simulink model "Solo_fast_2"  (R2024b)
settings: Solver=VariableStepAuto  StartTime=0.0  StopTime=86400*2  RelTol=1e-3
settings Model: Creator=Laura  LastModifiedBy=Laura

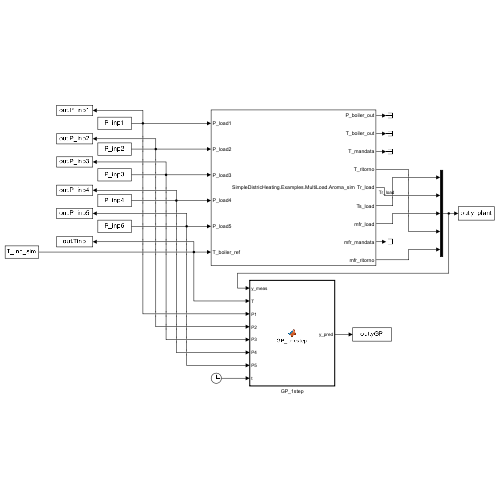
[thumbnail: Simulink's stored preview of the top-level diagram]
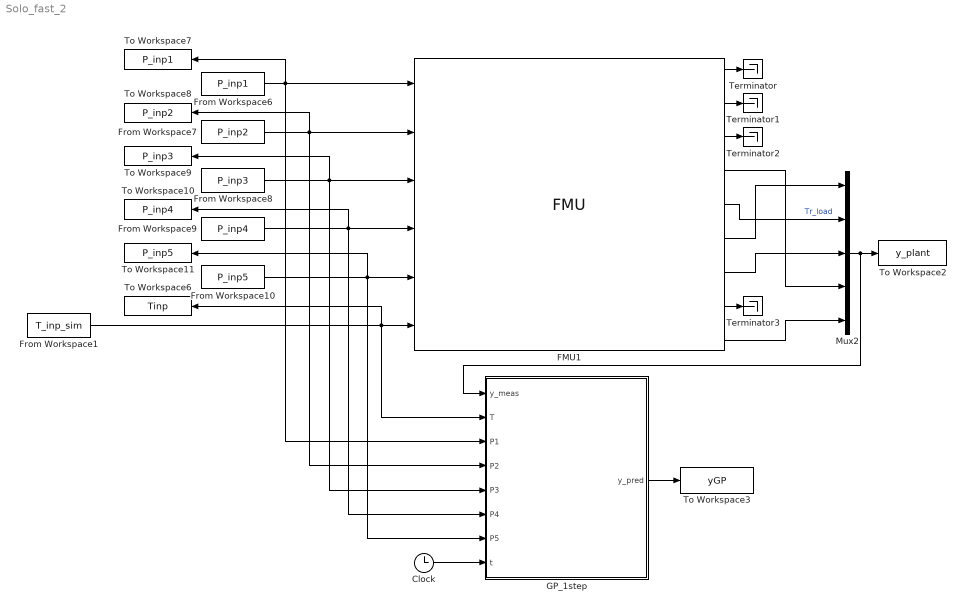
== system Solo_fast_2 ==
  Clock : Clock
  FMU1 : FMU  FMUName=SimpleDistricHeating.Examples.MultiLoad.Aroma_sim.fmu  FMUMode=ModelExchange  FMUInitializeEnumObject=off  boiler=struct('P_max',100000000.0,'P_min',1000.0,'T_vol',353.15,'V',0.16,'boilePowerUnit',struct('b',0.001),'boilerInsideVolume',struct('T_amb',288.15,'UA',0.0,'allowFlowReversal',boolean(false)),'boilerPIControl',struct('D',struct('y_start',0.0),'FFzero',struct('k',0.0),'Nd',10.0,'Ni',0.9,'P',struct('k',1.0),'Td',0.1,'Ti',8.0,'addD',struct('k2',-1.0),'addFF',struct('k1',1.0),'addI',struct('k1',1.0,'k2',-1.0,'k3',1.0),'addP',struct('k2',-1.0),'addPID',struct('k1',1.0,'k2',1.0,'k3',1.0),'addSat',struct('k1',1.0,'k2',-1.0),'k',50000.0,'kFF',1.0,'limiter',struct('uMax',100000000.0,'uMin',1000.0),'wd',0.0,'wp',1.0,'xd_start',0.0,'xi_start',0.0),'integralTime',16.0)  load1=struct('Kv',36.0,'dp_nom',400000.0,'load',struct('b',0.001),'loadValveControl',struct('Dzero',struct('k',0.0),'FFzero',struct('k',0.0),'Izero',struct('k',0.0),'Nd',10.0,'Ni',0.9,'P',struct('k',1.0),'Td',0.1,'Ti',0.5,'addFF',struct('k1',1.0),'addP',struct('k2',-1.0),'addPID',struct('k1',1.0,'k2',1.0,'k3',1.0),'k',0.05,'kFF',1.0,'limiter',struct('uMax',1.0,'uMin',0.0),'wd',0.0,'wp',1.0,'xd_start',0.0,'xi_start',0.0),'m_nom',25.0,'theta_min',0.001,'theta_nom',1.0)  load2=struct('Kv',36.0,'dp_nom',400000.0,'load',struct('b',0.001),'loadValveControl',struct('Dzero',struct('k',0.0),'FFzero',struct('k',0.0),'Izero',struct('k',0.0),'Nd',10.0,'Ni',0.9,'P',struct('k',1.0),'Td',0.1,'Ti',0.5,'addFF',struct('k1',1.0),'addP',struct('k2',-1.0),'addPID',struct('k1',1.0,'k2',1.0,'k3',1.0),'k',0.05,'kFF',1.0,'limiter',struct('uMax',1.0,'uMin',0.0),'wd',0.0,'wp',1.0,'xd_start',0.0,'xi_start',0.0),'m_nom',25.0,'theta_min',0.001,'theta_nom',1.0)  load3=struct('Kv',36.0,'dp_nom',400000.0,'load',struct('b',0.001),'loadValveControl',struct('Dzero',struct('k',0.0),'FFzero',struct('k',0.0),'Izero',struct('k',0.0),'Nd',10.0,'Ni',0.9,'P',struct('k',1.0),'Td',0.1,'Ti',0.5,'addFF',struct('k1',1.0),'addP',struct('k2',-1.0),'addPID',struct('k1',1.0,'k2',1.0,'k3',1.0),'k',0.05,'kFF',1.0,'limiter',struct('uMax',1.0,'uMin',0.0),'wd',0.0,'wp',1.0,'xd_start',0.0,'xi_start',0.0),'m_nom',25.0,'theta_min',0.001,'theta_nom',1.0)  load4=struct('Kv',36.0,'dp_nom',400000.0,'load',struct('b',0.001),'loadValveControl',struct('Dzero',struct('k',0.0),'FFzero',struct('k',0.0),'Izero',struct('k',0.0),'Nd',10.0,'Ni',0.9,'P',struct('k',1.0),'Td',0.1,'Ti',0.5,'addFF',struct('k1',1.0),'addP',struct('k2',-1.0),'addPID',struct('k1',1.0,'k2',1.0,'k3',1.0),'k',0.05,'kFF',1.0,'limiter',struct('uMax',1.0,'uMin',0.0),'wd',0.0,'wp',1.0,'xd_start',0.0,'xi_start',0.0),'m_nom',25.0,'theta_min',0.001,'theta_nom',1.0)  load5=struct('Kv',36.0,'dp_nom',400000.0,'load',struct('b',0.001),'loadValveControl',struct('Dzero',struct('k',0.0),'FFzero',struct('k',0.0),'Izero',struct('k',0.0),'Nd',10.0,'Ni',0.9,'P',struct('k',1.0),'Td',0.1,'Ti',0.5,'addFF',struct('k1',1.0),'addP',struct('k2',-1.0),'addPID',struct('k1',1.0,'k2',1.0,'k3',1.0),'k',0.05,'kFF',1.0,'limiter',struct('uMax',1.0,'uMin',0.0),'wd',0.0,'wp',1.0,'xd_start',0.0,'xi_start',0.0),'m_nom',25.0,'theta_min',0.001,'theta_nom',1.0)  load_ref=struct('k',65.0)  pressureAccumulator=struct('T0',338.15,'p_2',499999.9999999999)  pumpDifferentialPressure=struct('dp',499999.9999999999)  r10=struct('D',0.107,'L',500.0,'T_ext',298.15,'T_start',337.15,'cf',0.004,'conductivity_pipe_ins',0.02,'dIns',0.2,'dWall',0.003,'lambda',45.0,'rhomcm',3120000.0,'u_nom',1.5)  r21=struct('D',0.107,'L',282.8,'T_ext',298.15,'T_start',337.15,'cf',0.004,'conductivity_pipe_ins',0.02,'dIns',0.2,'dWall',0.003,'lambda',45.0,'rhomcm',3120000.0,'u_nom',1.5)  r32=struct('D',0.083,'L',500.0,'T_ext',298.15,'T_start',337.15,'cf',0.004,'conductivity_pipe_ins',0.02,'dIns',0.2,'dWall',0.003,'lambda',45.0,'rhomcm',3120000.0,'u_nom',1.5)  r43=struct('D',0.083,'L',282.8,'T_ext',298.15,'T_start',337.15,'cf',0.004,'conductivity_pipe_ins',0.02,'dIns',0.2,'dWall',0.003,'lambda',45.0,'rhomcm',3120000.0,'u_nom',1.5)  r54=struct('D',0.07000000000000001,'L',400.0,'T_ext',298.15,'T_start',337.15,'cf',0.004,'conductivity_pipe_ins',0.02,'dIns',0.2,'dWall',0.003,'lambda',45.0,'rhomcm',3120000.0,'u_nom',1.5)  r61=struct('D',0.107,'L',282.8,'T_ext',298.15,'T_start',337.15,'cf',0.004,'conductivity_pipe_ins',0.02,'dIns',0.2,'dWall',0.003,'lambda',45.0,'rhomcm',3120000.0,'u_nom',1.5)  r74=struct('D',0.083,'L',282.8,'T_ext',298.15,'T_start',337.15,'cf',0.004,'conductivity_pipe_ins',0.02,'dIns',0.2,'dWall',0.003,'lambda',45.0,'rhomcm',3120000.0,'u_nom',1.5)  r76=struct('D',0.083,'L',500.0,'T_ext',298.15,'T_start',337.15,'cf',0.004,'conductivity_pipe_ins',0.02,'dIns',0.2,'dWall',0.003,'lambda',45.0,'rhomcm',3120000.0,'u_nom',1.5)  r87=struct('D',0.07000000000000001,'L',600.0,'T_ext',298.15,'T_start',337.15,'cf',0.004,'conductivity_pipe_ins',0.02,'dIns',0.2,'dWall',0.003,'lambda',45.0,'rhomcm',3120000.0,'u_nom',1.5)  s01=struct('D',0.107,'L',500.0,'T_ext',298.15,'T_start',353.15,'cf',0.004,'conductivity_pipe_ins',0.02,'dIns',0.2,'dWall',0.003,'lambda',45.0,'rhomcm',3120000.0,'u_nom',1.5)  s12=struct('D',0.107,'L',282.8,'T_ext',298.15,'T_start',353.15,'cf',0.004,'conductivity_pipe_ins',0.02,'dIns',0.2,'dWall',0.003,'lambda',45.0,'rhomcm',3120000.0,'u_nom',1.5)  s16=struct('D',0.107,'L',282.8,'T_ext',298.15,'T_start',353.15,'cf',0.004,'conductivity_pipe_ins',0.02,'dIns',0.2,'dWall',0.003,'lambda',45.0,'rhomcm',3120000.0,'u_nom',1.5)  s23=struct('D',0.083,'L',500.0,'T_ext',298.15,'T_start',353.15,'cf',0.004,'conductivity_pipe_ins',0.02,'dIns',0.2,'dWall',0.003,'lambda',45.0,'rhomcm',3120000.0,'u_nom',1.5)  s34=struct('D',0.083,'L',282.8,'T_ext',298.15,'T_start',353.15,'cf',0.004,'conductivity_pipe_ins',0.02,'dIns',0.2,'dWall',0.003,'lambda',45.0,'rhomcm',3120000.0,'u_nom',1.5)  s45=struct('D',0.07000000000000001,'L',400.0,'T_ext',298.15,'T_start',353.15,'cf',0.004,'conductivity_pipe_ins',0.02,'dIns',0.2,'dWall',0.003,'lambda',45.0,'rhomcm',3120000.0,'u_nom',1.5)  s47=struct('D',0.083,'L',282.8,'T_ext',298.15,'T_start',353.15,'cf',0.004,'conductivity_pipe_ins',0.02,'dIns',0.2,'dWall',0.003,'lambda',45.0,'rhomcm',3120000.0,'u_nom',1.5)  s67=struct('D',0.083,'L',500.0,'T_ext',298.15,'T_start',353.15,'cf',0.004,'conductivity_pipe_ins',0.02,'dIns',0.2,'dWall',0.003,'lambda',45.0,'rhomcm',3120000.0,'u_nom',1.5)  s78=struct('D',0.07000000000000001,'L',600.0,'T_ext',298.15,'T_start',353.15,'cf',0.004,'conductivity_pipe_ins',0.02,'dIns',0.2,'dWall',0.003,'lambda',45.0,'rhomcm',3120000.0,'u_nom',1.5)  mask(SimpleDistricHeating.Examples.MultiLoad.Aroma_sim [Model Exchange, v2.0]){}
      settings: MultithreadedSim=off
      mask Display:
      | disp('SimpleDistricHeating.Examples.MultiLoad.Aroma_sim');
      | port_label('output',1,'P_boiler_out');
      | port_label('output',2,'T_boiler_out');
      | port_label('output',3,'T_mandata');
      | port_label('output',4,'T_ritorno');
      | port_label('output',5,'Tr_load');
      | port_label('output',6,'Ts_load');
      | port_label('output',7,'mfr_load');
      | port_label('output',8,'mfr_mandata');
      | port_label('output',9,'mfr_ritorno');
      | port_label('input',1,'P_load1');
      | port_label('input',2,'P_load2');
      | port_label('input',3,'P_load3');
      | port_label('input',4,'P_load4');
      | port_label('input',5,'P_load5');
      | port_label('input',6,'T_boiler_ref');
  From Workspace1 : FromWorkspace  VariableName=T_inp_sim  SampleTime=-1
  From Workspace10 : FromWorkspace  VariableName=P_inp5  SampleTime=-1
  From Workspace6 : FromWorkspace  VariableName=P_inp1  SampleTime=-1
  From Workspace7 : FromWorkspace  VariableName=P_inp2  SampleTime=-1
  From Workspace8 : FromWorkspace  VariableName=P_inp3  SampleTime=-1
  From Workspace9 : FromWorkspace  VariableName=P_inp4  SampleTime=-1
  GP_1step : MATLAB Function  TreatAsAtomicUnit=on  SystemSampleTime=300
  Mux2 : Mux  Inputs=5
  Terminator{,1..3} (4 alike) : Terminator
  To Workspace10 : ToWorkspace  VariableName=P_inp4  SampleTime=300
  To Workspace11 : ToWorkspace  VariableName=P_inp5  SampleTime=300
  To Workspace2 : ToWorkspace  VariableName=y_plant  SampleTime=300
  To Workspace3 : ToWorkspace  VariableName=yGP  SampleTime=300
  To Workspace6 : ToWorkspace  VariableName=Tinp  SampleTime=300
  To Workspace7 : ToWorkspace  VariableName=P_inp1  SampleTime=300
  To Workspace8 : ToWorkspace  VariableName=P_inp2  SampleTime=300
  To Workspace9 : ToWorkspace  VariableName=P_inp3  SampleTime=300
  wires:
  Mux2/1 -> GP_1step/1(y_meas), To Workspace2/1
  From Workspace9/1 -> FMU1/4, GP_1step/6(P4), To Workspace10/1
  From Workspace1/1 -> FMU1/6, GP_1step/2(T), To Workspace6/1
  GP_1step/1(y_pred) -> To Workspace3/1
  Clock/1 -> GP_1step/8(t)
  From Workspace6/1 -> FMU1/1, GP_1step/3(P1), To Workspace7/1
  From Workspace8/1 -> FMU1/3, GP_1step/5(P3), To Workspace9/1
  From Workspace10/1 -> FMU1/5, GP_1step/7(P5), To Workspace11/1
  From Workspace7/1 -> FMU1/2, GP_1step/4(P2), To Workspace8/1
  FMU1/1 -> Terminator/1
  FMU1/2 -> Terminator1/1
  FMU1/3 -> Terminator2/1
  FMU1/4 -> Mux2/4
  FMU1/9 -> Mux2/5
  FMU1/8 -> Terminator3/1
  FMU1/6 -> Mux2/1
  FMU1/5 -> Mux2/2  "Tr_load"
  FMU1/7 -> Mux2/3

== matlab function Solo_fast_2/GP_1step ==
  data: y_pred output; y_meas input; T input; P1 input; P2 input; P3 input; P4 input; P5 input; t input
function y_pred = GP_onestep(y_meas, T, P1, P2, P3, P4, P5, t)
    
    % Declare we use some matlab function inside the Simulink block
    coder.extrinsic('fitrgp', 'predict')
    
    % Declare parameters
    n_regression = 4;
    sampling_time = 300;
    n_input = 6;
    n_output = 17;
    n_max = 48; %300

    % Declare persistent variables whose dimension is not fixed (used to have an increasing dataset)
    persistent u_pers u_stack y_pred_tot y_pers y_stack_1 y_stack_2 y_stack_3 y_stack_4 y_stack_5 y_stack_6 y_stack_7 y_stack_8 y_stack_9 y_stack_10 y_stack_11 y_stack_12 y_stack_13 y_stack_14 y_stack_15 y_stack_16 y_stack_17
    coder.varsize('u_pers', [inf, n_input]);
    coder.varsize('u_stack', [inf, n_input*n_regression]);
    coder.varsize('y_pred_tot', [inf, n_output]);
    coder.varsize('y_pers', [inf, n_output]);
    coder.varsize('y_stack_1', [inf, n_regression]);
    coder.varsize('y_stack_2', [inf, n_regression]);
    coder.varsize('y_stack_3', [inf, n_regression]);
    coder.varsize('y_stack_4', [inf, n_regression]);
    coder.varsize('y_stack_5', [inf, n_regression]);
    coder.varsize('y_stack_6', [inf, n_regression]);
    coder.varsize('y_stack_7', [inf, n_regression]);
    coder.varsize('y_stack_8', [inf, n_regression]);
    coder.varsize('y_stack_9', [inf, n_regression]);
    coder.varsize('y_stack_10', [inf, n_regression]);
    coder.varsize('y_stack_11', [inf, n_regression]);
    coder.varsize('y_stack_12', [inf, n_regression]);
    coder.varsize('y_stack_13', [inf, n_regression]);
    coder.varsize('y_stack_14', [inf, n_regression]);
    coder.varsize('y_stack_15', [inf, n_regression]);
    coder.varsize('y_stack_16', [inf, n_regression]);
    coder.varsize('y_stack_17', [inf, n_regression]);
    
    % Initialize persistent variables
    if isempty(u_pers)
        u_pers = zeros(1,n_input);
        u_stack = zeros(1,n_input*n_regression);
        y_pred_tot = zeros(1,n_output);
        y_pers = zeros(1,n_output);
        y_stack_1 = zeros(1,n_regression);
        y_stack_2 = zeros(1,n_regression);
        y_stack_3 = zeros(1,n_regression);
        y_stack_4 = zeros(1,n_regression);
        y_stack_5 = zeros(1,n_regression);
        y_stack_6 = zeros(1,n_regression);
        y_stack_7 = zeros(1,n_regression);
        y_stack_8 = zeros(1,n_regression);
        y_stack_9 = zeros(1,n_regression);
        y_stack_10 = zeros(1,n_regression);
        y_stack_11 = zeros(1,n_regression);
        y_stack_12 = zeros(1,n_regression);
        y_stack_13 = zeros(1,n_regression);
        y_stack_14 = zeros(1,n_regression);
        y_stack_15 = zeros(1,n_regression);
        y_stack_16 = zeros(1,n_regression);
        y_stack_17 = zeros(1,n_regression);
    end
    
    % Output initialization
    y_pred = zeros(17,1);

    % Create increasing input dataset
    u_new = [T P1 P2 P3 P4 P5];
    u_pers = [u_pers; u_new];
    
    % Create increasing output dataset
    y_meas = [y_meas(1); y_meas(6); y_meas(11); y_meas(4); y_meas(9); y_meas(14); y_meas(2); y_meas(7); y_meas(12); y_meas(3); y_meas(8); y_meas(13); y_meas(5); y_meas(10); y_meas(15); y_meas(16); y_meas(17)];
    y_pers = [y_pers; y_meas.'];
    
    % Remove first row of zeros
    if u_pers(1,1) == 0
        u_pers = u_pers(2:end,:);
        y_pers = y_pers(2:end,:);
    end
    
    % Start to build GP when data are at least n_regression
    if t >= sampling_time*n_regression

        % Build the regressive variables
        u_regr = zeros(1,size(u_stack,2));
        u_regr_test = zeros(1,size(u_stack,2));
        k = 1;
        for i = 1:n_regression
            u_regr(1,k:k+n_input-1) = u_pers(end-i,:);
            u_regr_test(1,k:k+n_input-1) = u_pers(end-i+1,:);
            k = k + n_input;
        end

        y_regr_1 = zeros(1,size(y_stack_1,2));
        y_regr_1_test = zeros(1,size(y_stack_1,2));
        y_regr_2 = zeros(1,size(y_stack_2,2));
        y_regr_2_test = zeros(1,size(y_stack_2,2));
        y_regr_3 = zeros(1,size(y_stack_3,2));
        y_regr_3_test = zeros(1,size(y_stack_3,2));
        y_regr_4 = zeros(1,size(y_stack_4,2));
        y_regr_4_test = zeros(1,size(y_stack_4,2));
        y_regr_5 = zeros(1,size(y_stack_5,2));
        y_regr_5_test = zeros(1,size(y_stack_5,2));
        y_regr_6 = zeros(1,size(y_stack_6,2));
        y_regr_6_test = zeros(1,size(y_stack_6,2));
        y_regr_7 = zeros(1,size(y_stack_7,2));
        y_regr_7_test = zeros(1,size(y_stack_7,2));
        y_regr_8 = zeros(1,size(y_stack_8,2));
        y_regr_8_test = zeros(1,size(y_stack_8,2));
        y_regr_9 = zeros(1,size(y_stack_9,2));
        y_regr_9_test = zeros(1,size(y_stack_9,2));
        y_regr_10 = zeros(1,size(y_stack_10,2));
        y_regr_10_test = zeros(1,size(y_stack_10,2));
        y_regr_11 = zeros(1,size(y_stack_11,2));
        y_regr_11_test = zeros(1,size(y_stack_11,2));
        y_regr_12 = zeros(1,size(y_stack_12,2));
        y_regr_12_test = zeros(1,size(y_stack_12,2));
        y_regr_13 = zeros(1,size(y_stack_13,2));
        y_regr_13_test = zeros(1,size(y_stack_13,2));
        y_regr_14 = zeros(1,size(y_stack_14,2));
        y_regr_14_test = zeros(1,size(y_stack_14,2));
        y_regr_15 = zeros(1,size(y_stack_15,2));
        y_regr_15_test = zeros(1,size(y_stack_15,2));
        y_regr_16 = zeros(1,size(y_stack_16,2));
        y_regr_16_test = zeros(1,size(y_stack_16,2));
        y_regr_17 = zeros(1,size(y_stack_17,2));
        y_regr_17_test = zeros(1,size(y_stack_17,2));

        for i = 1:n_regression
            y_regr_1(1,i) = y_pers(end-i,1);
            y_regr_1_test(1,i) = y_pers(end-i+1,1);
            y_regr_2(1,i) = y_pers(end-i,2);
            y_regr_2_test(1,i) = y_pers(end-i+1,2);
            y_regr_3(1,i) = y_pers(end-i,3);
            y_regr_3_test(1,i) = y_pers(end-i+1,3);
            y_regr_4(1,i) = y_pers(end-i,4);
            y_regr_4_test(1,i) = y_pers(end-i+1,4);
            y_regr_5(1,i) = y_pers(end-i,5);
            y_regr_5_test(1,i) = y_pers(end-i+1,5);
            y_regr_6(1,i) = y_pers(end-i,6);
            y_regr_6_test(1,i) = y_pers(end-i+1,6);
            y_regr_7(1,i) = y_pers(end-i,7);
            y_regr_7_test(1,i) = y_pers(end-i+1,7);
            y_regr_8(1,i) = y_pers(end-i,8);
            y_regr_8_test(1,i) = y_pers(end-i+1,8);
            y_regr_9(1,i) = y_pers(end-i,9);
            y_regr_9_test(1,i) = y_pers(end-i+1,9);
            y_regr_10(1,i) = y_pers(end-i,10);
            y_regr_10_test(1,i) = y_pers(end-i+1,10);
            y_regr_11(1,i) = y_pers(end-i,11);
            y_regr_11_test(1,i) = y_pers(end-i+1,11);
            y_regr_12(1,i) = y_pers(end-i,12);
            y_regr_12_test(1,i) = y_pers(end-i+1,12);
            y_regr_13(1,i) = y_pers(end-i,13);
            y_regr_13_test(1,i) = y_pers(end-i+1,13);
            y_regr_14(1,i) = y_pers(end-i,14);
            y_regr_14_test(1,i) = y_pers(end-i+1,14);
            y_regr_15(1,i) = y_pers(end-i,15);
            y_regr_15_test(1,i) = y_pers(end-i+1,15);
            y_regr_16(1,i) = y_pers(end-i,16);
            y_regr_16_test(1,i) = y_pers(end-i+1,16);
            y_regr_17(1,i) = y_pers(end-i,17);
            y_regr_17_test(1,i) = y_pers(end-i+1,17);
        end
    
        % Stack vertically
        u_stack = [u_stack; u_regr];
        y_stack_1 = [y_stack_1; y_regr_1];
        y_stack_2 = [y_stack_2; y_regr_2];
        y_stack_3 = [y_stack_3; y_regr_3];
        y_stack_4 = [y_stack_4; y_regr_4];
        y_stack_5 = [y_stack_5; y_regr_5];
        y_stack_6 = [y_stack_6; y_regr_6];
        y_stack_7 = [y_stack_7; y_regr_7];
        y_stack_8 = [y_stack_8; y_regr_8];
        y_stack_9 = [y_stack_9; y_regr_9];
        y_stack_10 = [y_stack_10; y_regr_10];
        y_stack_11 = [y_stack_11; y_regr_11];
        y_stack_12 = [y_stack_12; y_regr_12];
        y_stack_13 = [y_stack_13; y_regr_13];
        y_stack_14 = [y_stack_14; y_regr_14];
        y_stack_15 = [y_stack_15; y_regr_15];
        y_stack_16 = [y_stack_16; y_regr_16];
        y_stack_17 = [y_stack_17; y_regr_17];
               
        %%%%%%%%%% Input of GP %%%%%%%%%%
        x_1 = [y_stack_1 u_stack];
        x_2 = [y_stack_2 u_stack];
        x_3 = [y_stack_3 u_stack];
        x_4 = [y_stack_4 u_stack];
        x_5 = [y_stack_5 u_stack];
        x_6 = [y_stack_6 u_stack];
        x_7 = [y_stack_7 u_stack];
        x_8 = [y_stack_8 u_stack];
        x_9 = [y_stack_9 u_stack];
        x_10 = [y_stack_10 u_stack];
        x_11 = [y_stack_11 u_stack];
        x_12 = [y_stack_12 u_stack];
        x_13 = [y_stack_13 u_stack];
        x_14 = [y_stack_14 u_stack];
        x_15 = [y_stack_15 u_stack];
        x_16 = [y_stack_16 u_stack];
        x_17 = [y_stack_17 u_stack];


        %%%%%%%%%% GP model learning, for each output %%%%%%%%%%
        gpr_model1 = fitrgp(x_1, y_pers(n_regression:end,1));
        gpr_model2 = fitrgp(x_2, y_pers(n_regression:end,2));
        gpr_model3 = fitrgp(x_3, y_pers(n_regression:end,3));
        gpr_model4 = fitrgp(x_4, y_pers(n_regression:end,4));
        gpr_model5 = fitrgp(x_5, y_pers(n_regression:end,5));
        gpr_model6 = fitrgp(x_6, y_pers(n_regression:end,6));
        gpr_model7 = fitrgp(x_7, y_pers(n_regression:end,7));
        gpr_model8 = fitrgp(x_8, y_pers(n_regression:end,8));
        gpr_model9 = fitrgp(x_9, y_pers(n_regression:end,9));
        gpr_model10 = fitrgp(x_10, y_pers(n_regression:end,10));
        gpr_model11 = fitrgp(x_11, y_pers(n_regression:end,11));
        gpr_model12 = fitrgp(x_12, y_pers(n_regression:end,12));
        gpr_model13 = fitrgp(x_13, y_pers(n_regression:end,13));
        gpr_model14 = fitrgp(x_14, y_pers(n_regression:end,14));
        gpr_model15 = fitrgp(x_15, y_pers(n_regression:end,15));
        gpr_model16 = fitrgp(x_16, y_pers(n_regression:end,16));
        gpr_model17 = fitrgp(x_17, y_pers(n_regression:end,17));
        
        %%%%%%%%%% GP prediction %%%%%%%%%%
        y_pred(1) = predict(gpr_model1, [y_regr_1_test u_regr_test]);
        y_pred(2) = predict(gpr_model2, [y_regr_2_test u_regr_test]);
        y_pred(3) = predict(gpr_model3, [y_regr_3_test u_regr_test]);
        y_pred(4) = predict(gpr_model4, [y_regr_4_test u_regr_test]);
        y_pred(5) = predict(gpr_model5, [y_regr_5_test u_regr_test]);
        y_pred(6) = predict(gpr_model6, [y_regr_6_test u_regr_test]);
        y_pred(7) = predict(gpr_model7, [y_regr_7_test u_regr_test]);
        y_pred(8) = predict(gpr_model8, [y_regr_8_test u_regr_test]);
        y_pred(9) = predict(gpr_model9, [y_regr_9_test u_regr_test]);
        y_pred(10) = predict(gpr_model10, [y_regr_10_test u_regr_test]);
        y_pred(11) = predict(gpr_model11, [y_regr_11_test u_regr_test]);
        y_pred(12) = predict(gpr_model12, [y_regr_12_test u_regr_test]);
        y_pred(13) = predict(gpr_model13, [y_regr_13_test u_regr_test]);
        y_pred(14) = predict(gpr_model14, [y_regr_14_test u_regr_test]);
        y_pred(15) = predict(gpr_model15, [y_regr_15_test u_regr_test]);
        y_pred(16) = predict(gpr_model16, [y_regr_16_test u_regr_test]);
        y_pred(17) = predict(gpr_model17, [y_regr_17_test u_regr_test]);
       
        y_pred_tot = [y_pred_tot; y_pred.'];
    
        %%%%%%%%%% Limit the size of GP %%%%%%%%%%
        if size(u_stack,1) > n_max
            u_stack = u_stack(end-n_max:end,:);
            u_pers = u_pers(end-n_max-n_regression+1:end,:);
            y_pred_tot = y_pred_tot(end-n_max:end,:);
            y_pers = y_pers(end-n_max-n_regression+1:end,:);
            y_stack_1 = y_stack_1(end-n_max:end,:);
            y_stack_2 = y_stack_2(end-n_max:end,:);
            y_stack_3 = y_stack_3(end-n_max:end,:);
            y_stack_4 = y_stack_4(end-n_max:end,:);
            y_stack_5 = y_stack_5(end-n_max:end,:);
            y_stack_6 = y_stack_6(end-n_max:end,:);
            y_stack_7 = y_stack_7(end-n_max:end,:);
            y_stack_8 = y_stack_8(end-n_max:end,:);
            y_stack_9 = y_stack_9(end-n_max:end,:);
            y_stack_10 = y_stack_10(end-n_max:end,:);
            y_stack_11 = y_stack_11(end-n_max:end,:);
            y_stack_12 = y_stack_12(end-n_max:end,:);
            y_stack_13 = y_stack_13(end-n_max:end,:);
            y_stack_14 = y_stack_14(end-n_max:end,:);
            y_stack_15 = y_stack_15(end-n_max:end,:);
            y_stack_16 = y_stack_16(end-n_max:end,:);
            y_stack_17 = y_stack_17(end-n_max:end,:);
        end
    end
end
